simulink model "sampleModel1656"  (R2023a)
settings: Solver=VariableStepAuto  StartTime=0.0  StopTime=10.0  RelTol=1e-3
libraries: hdlsllib x6, simulink x1
settings Model: Creator=user1  LastModifiedBy=user1

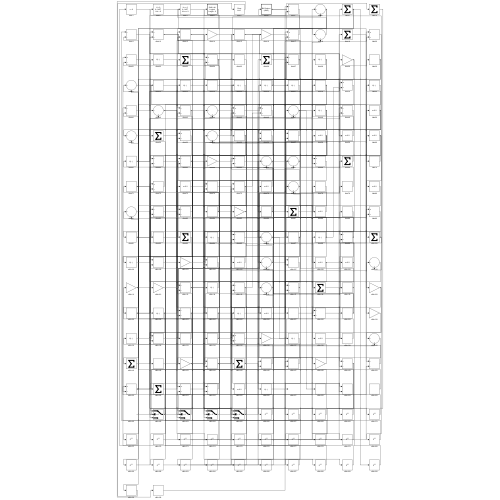
[thumbnail: Simulink's stored preview of the top-level diagram]
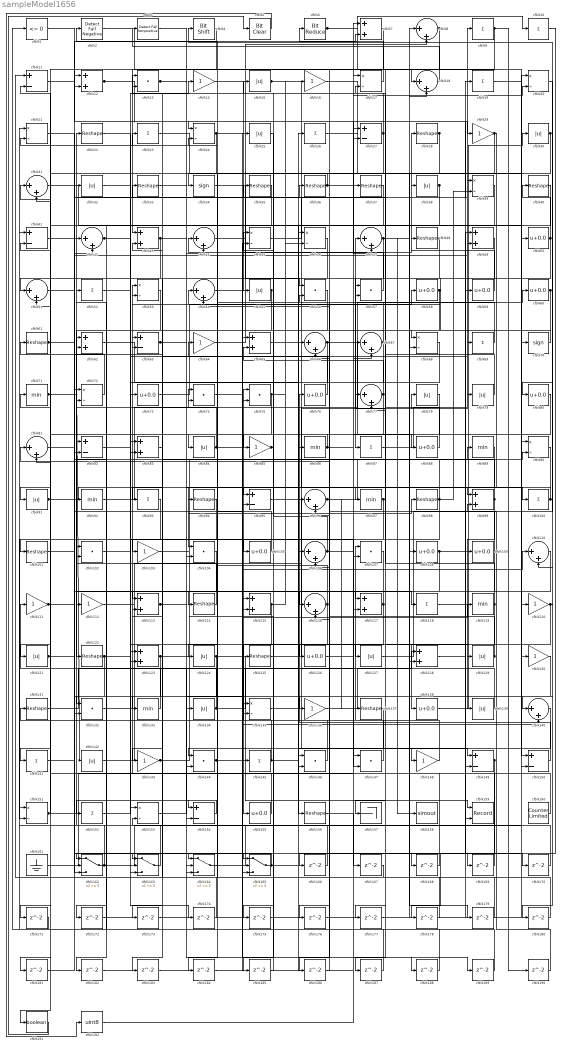
== system sampleModel1656 ==
  cfblk1 : hdlsllib/Logic and Bit Operations/Compare To Zero  relop=<=  OutDataTypeStr=boolean
  cfblk{9..10,19,23,26,52,69,87,93,100,118,141,145,152} (14 alike) : Sum  Inputs=+
  cfblk{22,28,33,35..37,40,48,61,94,98,101,114,122,125,131,137,156} (18 alike) : Reshape
  cfblk{13,56..57,74..75,102,104,107,132,144,146..147} (12 alike) : DotProduct  OutDataTypeStr=Inherit: Inherit via internal rule
  cfblk{14,16,29,64,85,103,111..112,120,130,136,143,148} (13 alike) : Gain
  cfblk{50,58..60,73,76,80,88,105,108..109,126,138,155} (14 alike) : Bias  Bias=0.0  SaturateOnIntegerOverflow=off
  cfblk{8,18,31,42,44,47,51,54,66..67,77,81,96,106,110,116,140} (17 alike) : Sum  Inputs=|++
  cfblk{11,27,41,63,82,95,149..150,154} (9 alike) : Sum  Inputs=+-
  cfblk{7,12,43,49,62,65,83,99,113,115,117,123,128} (13 alike) : Sum
  cfblk{71,86,89,92,97,119,133} (7 alike) : MinMax
  cfblk{15,25,30,32,38,55,78..79,84,91,121,124,127,129,134,139,142} (17 alike) : Abs  SaturateOnIntegerOverflow=off
  cfblk{17,20..21,24,39,45..46,53,68,72,90,135,151,153} (14 alike) : Product  Inputs=*/  RndMeth=Zero  SaturateOnIntegerOverflow=on
  cfblk157 : Terminator
  cfblk158 : ToWorkspace  VariableName=simout  SaveFormat=Timeseries  SampleTime=-1
  cfblk159 : Record  FileSettingsInternal="{\"entries\":[{\"content\":{\"excelSettings\":{\"content\":{},\"type\":\"Streamout.ExcelSettings\"}},\"type\":\"Streamout.FileSettingStorage\",\"uuid\":\"\"}],\"packageUris\":[\"http:\\/\\/schema.mathworks.com\\/mf0\\/streamout_blocks\\/R2020a\"],\"version\":\"1.0\"}"  Layout=[1 1]  SignalsInternal="{\"entries\":[{\"content\":{\"signals\":[{\"content\":{\"blockPath\":[],\"dimensions\":[1],\"domain\":\"\",\"lineColor\":\"#a2142f\",\"plots\":[1],\"port\":1,\"signalID\":2593,\"signalName\":\"XY Graph:1\"},\"type\":\"RecordBlkView.Signal\",\"uuid\":\"\"},{\"content\":{\"blockPath\":[],\"dimensions\":[1],\"domain\":\"\",\"lineColor\":\"#139fff\",\"plots\":[1],\"port\":2,\"signalID\":2596,\"signalName\":\"XY Graph:2\"},\"type\":\"RecordBlkView.Signal\",\"uuid\":\"\"}]},\"type\":\"RecordBlkView.InputSignals\",\"uuid\":\"\"}],\"packageUris\":[\"http:\\/\\/schema.mathworks.com\\/mf0\\/streamout_blocks\\/R2020a\"],\"version\":\"1.0\"}"  VisualizationBindings="{\"xyplotplugin\":{\"info\":[{\"series\":[{\"bindingParametersList\":[{\"parameter\":\"X-Axis\",\"signalID\":2593,\"signalName\":\"XY Graph:1\"},{\"parameter\":\"Y-Axis\",\"signalID\":2596,\"signalName\":\"XY Graph:2\"}],\"seriesID\":62182}],\"subplotID\":1}]}}"  CompatibilityTag=XY  st=-1
  cfblk160 : hdlsllib/Sources/Counter Limited  uplimit=7  tsamp=-1
  cfblk161 : Ground
  cfblk{162..165} (4 alike) : Switch  SaturateOnIntegerOverflow=off  InputSameDT=off
  cfblk{166..190} (25 alike) : Delay  SampleTime=1
  cfblk191 : DataTypeConversion  OutDataTypeStr=boolean  SaturateOnIntegerOverflow=off  RndMeth=Floor
  cfblk192 : DataTypeConversion  OutDataTypeStr=uint8  SaturateOnIntegerOverflow=off  RndMeth=Floor
  cfblk2 : hdlsllib/Logic and Bit Operations/Detect Fall Negative  vinit=0  OutDataTypeStr=boolean
  cfblk3 : hdlsllib/Logic and Bit Operations/Detect Fall Nonpositive  vinit=0  OutDataTypeStr=boolean
  cfblk34 : Signum
  cfblk4 : hdlsllib/Logic and Bit Operations/Bit Shift  mode=Shift Left Logical  N=0
  cfblk5 : simulink/Logic and Bit Operations/Bit Clear  iBit=0
      settings: LibrarySourceBlock=|
      | hdlsllib/Logic and Bit
      | Operations/Bit Clear
  cfblk6 : hdlsllib/Logic and Bit Operations/Bit Reduce  mode=AND
  cfblk70 : Signum
  wires:
  cfblk15/1 -> cfblk100/1, cfblk59/1
  cfblk13/1 -> cfblk165/1, cfblk189/1
  cfblk160/1 -> cfblk53/1
  cfblk150/1 -> cfblk76/1
  cfblk124/1 -> cfblk159/1, cfblk162/3
  cfblk103/1 -> cfblk98/1
  cfblk50/1 -> cfblk87/1, cfblk68/1, cfblk40/1, cfblk163/3
  cfblk59/1 -> cfblk28/1
  cfblk162/1 -> cfblk22/1, cfblk18/2
  cfblk46/1 -> cfblk103/1
  cfblk118/1 -> cfblk4/1
  cfblk101/1 -> cfblk12/1
  cfblk138/1 -> cfblk30/1
  cfblk143/1 -> cfblk89/1, cfblk125/1
  cfblk36/1 -> cfblk34/1, cfblk20/2
  cfblk149/1 -> cfblk177/1, cfblk178/1
  cfblk148/1 -> cfblk107/1
  cfblk125/1 -> cfblk78/1
  cfblk6/1 -> cfblk10/1, cfblk18/1
  cfblk127/1 -> cfblk50/1
  cfblk27/1 -> cfblk144/1, cfblk96/2, cfblk13/2
  cfblk142/1 -> cfblk66/1
  cfblk73/1 -> cfblk58/1
  cfblk41/1 -> cfblk12/2
  cfblk71/1 -> cfblk142/1, cfblk118/1
  cfblk55/1 -> cfblk122/1, cfblk163/1
  cfblk20/1 -> cfblk80/1
  cfblk19/1 -> cfblk70/1
  cfblk104/1 -> cfblk114/1
  cfblk96/1 -> cfblk20/1, cfblk137/1
  cfblk113/1 -> cfblk127/1, cfblk165/2
  cfblk120/1 -> cfblk138/1, cfblk180/1
  cfblk9/1 -> cfblk43/1, cfblk117/1, cfblk190/1
  cfblk163/1 -> cfblk52/1
  cfblk91/1 -> cfblk97/1, cfblk95/2
  cfblk64/1 -> cfblk8/2
  cfblk161/1 -> cfblk73/1
  cfblk95/1 -> cfblk148/1
  cfblk76/1 -> cfblk23/1
  cfblk117/1 -> cfblk112/1, cfblk185/1
  cfblk21/1 -> cfblk42/1
  cfblk147/1 -> cfblk75/1
  cfblk99/1 -> cfblk139/1, cfblk45/1, cfblk63/2
  cfblk112/1 -> cfblk60/1
  cfblk53/1 -> cfblk62/1
  cfblk116/1 -> cfblk155/1, cfblk74/2
  cfblk58/1 -> cfblk53/2, cfblk164/1, cfblk68/2, cfblk164/3
  cfblk67/1 -> cfblk2/1, cfblk124/1
  cfblk87/1 -> cfblk9/1
  cfblk31/1 -> cfblk150/1
  cfblk102/1 -> cfblk126/1
  cfblk25/1 -> cfblk85/1
  cfblk132/1 -> cfblk79/1
  cfblk42/1 -> cfblk153/1, cfblk107/2
  cfblk23/1 -> cfblk120/1
  cfblk57/1 -> cfblk44/1
  cfblk51/1 -> cfblk49/2
  cfblk98/1 -> cfblk147/2, cfblk77/1, cfblk66/2, cfblk39/2
  cfblk47/1 -> cfblk162/2, cfblk158/1, cfblk179/1
  cfblk12/1 -> cfblk55/1, cfblk47/2
  cfblk79/1 -> cfblk54/1
  cfblk65/1 -> cfblk86/1
  cfblk61/1 -> cfblk38/1, cfblk7/2
  cfblk24/1 -> cfblk21/2, cfblk82/2, cfblk140/2
  cfblk137/1 -> cfblk154/1
  cfblk17/1 -> cfblk6/1
  cfblk133/1 -> cfblk111/1
  cfblk11/1 -> cfblk29/1
  cfblk3/1 -> cfblk44/2
  cfblk8/1 -> cfblk136/1, cfblk51/2
  cfblk33/1 -> cfblk116/1
  cfblk121/1 -> cfblk33/1, cfblk63/1
  cfblk134/1 -> cfblk61/1, cfblk67/2
  cfblk153/1 -> cfblk134/1
  cfblk152/1 -> cfblk69/1
  cfblk89/1 -> cfblk104/1
  cfblk83/1 -> cfblk13/1
  cfblk135/1 -> cfblk149/1
  cfblk44/1 -> cfblk156/1
  cfblk52/1 -> cfblk14/1
  cfblk34/1 -> cfblk96/1
  cfblk62/1 -> cfblk106/1
  cfblk164/1 -> cfblk90/1
  cfblk86/1 -> cfblk84/1, cfblk88/1
  cfblk30/1 -> cfblk105/1, cfblk51/1
  cfblk4/1 -> cfblk101/1
  cfblk92/1 -> cfblk47/1
  cfblk88/1 -> cfblk32/1
  cfblk115/1 -> cfblk145/1, cfblk46/2
  cfblk16/1 -> cfblk149/2
  cfblk82/1 -> cfblk123/1
  cfblk131/1 -> cfblk17/1
  cfblk151/1 -> cfblk27/1, cfblk90/2, cfblk31/2
  cfblk136/1 -> cfblk128/1
  cfblk154/1 -> cfblk152/1
  cfblk32/1 -> cfblk83/1
  cfblk1/1 -> cfblk24/1
  cfblk69/1 -> cfblk17/2
  cfblk56/1 -> cfblk113/1
  cfblk105/1 -> cfblk74/1
  cfblk90/1 -> cfblk154/2
  cfblk77/1 -> cfblk92/1, cfblk65/2
  cfblk84/1 -> cfblk62/2, cfblk188/1
  cfblk68/1 -> cfblk83/2
  cfblk66/1 -> cfblk108/1, cfblk143/1
  cfblk49/1 -> cfblk133/1
  cfblk28/1 -> cfblk57/1, cfblk164/2
  cfblk122/1 -> cfblk36/1, cfblk132/2
  cfblk72/1 -> cfblk11/2
  cfblk119/1 -> cfblk157/1, cfblk77/2
  cfblk129/1 -> cfblk81/1, cfblk64/1
  cfblk37/1 -> cfblk81/2
  cfblk48/1 -> cfblk104/2, cfblk163/2, cfblk191/1
  cfblk146/1 -> cfblk71/1
  cfblk97/1 -> cfblk57/2, cfblk121/1, cfblk151/2
  cfblk109/1 -> cfblk54/2, cfblk117/2
  cfblk106/1 -> cfblk39/1, cfblk35/1
  cfblk7/1 -> cfblk56/1
  cfblk14/1 -> cfblk25/1
  cfblk45/1 -> cfblk19/1
  cfblk126/1 -> cfblk7/1
  cfblk111/1 -> cfblk41/2, cfblk165/3
  cfblk141/1 -> cfblk72/1
  cfblk2/1 -> cfblk130/1
  cfblk26/1 -> cfblk128/2
  cfblk43/1 -> cfblk91/1, cfblk168/1
  cfblk114/1 -> cfblk82/1
  cfblk165/1 -> cfblk26/1, cfblk162/1
  cfblk85/1 -> cfblk15/1, cfblk135/1
  cfblk35/1 -> cfblk132/1
  cfblk60/1 -> cfblk110/2, cfblk182/1, cfblk183/1
  cfblk39/1 -> cfblk146/2
  cfblk155/1 -> cfblk31/1
  cfblk18/1 -> cfblk3/1
  cfblk94/1 -> cfblk141/1
  cfblk144/1 -> cfblk119/1, cfblk110/1
  cfblk63/1 -> cfblk93/1, cfblk135/2
  cfblk54/1 -> cfblk48/1
  cfblk29/1 -> cfblk99/1, cfblk123/2
  cfblk75/1 -> cfblk102/1, cfblk16/1
  cfblk40/1 -> cfblk144/2
  cfblk108/1 -> cfblk109/1, cfblk186/1
  cfblk100/1 -> cfblk95/1, cfblk140/1
  cfblk123/1 -> cfblk45/2, cfblk172/1
  cfblk70/1 -> cfblk67/1
  cfblk139/1 -> cfblk115/1
  cfblk145/1 -> cfblk159/2, cfblk131/1
  cfblk74/1 -> cfblk129/1
  cfblk38/1 -> cfblk94/1, cfblk116/2
  cfblk10/1 -> cfblk166/1
  cfblk166/1 -> cfblk21/1
  cfblk156/1 -> cfblk167/1
  cfblk167/1 -> cfblk11/1
  cfblk168/1 -> cfblk56/2
  cfblk81/1 -> cfblk169/1
  cfblk169/1 -> cfblk43/2
  cfblk128/1 -> cfblk170/1
  cfblk170/1 -> cfblk153/2
  cfblk80/1 -> cfblk171/1
  cfblk171/1 -> cfblk1/1
  cfblk172/1 -> cfblk75/2
  cfblk130/1 -> cfblk173/1
  cfblk173/1 -> cfblk150/2
  cfblk22/1 -> cfblk174/1
  cfblk174/1 -> cfblk113/2
  cfblk107/1 -> cfblk175/1
  cfblk175/1 -> cfblk49/1
  cfblk140/1 -> cfblk176/1
  cfblk176/1 -> cfblk147/1
  cfblk177/1 -> cfblk8/1
  cfblk178/1 -> cfblk72/2
  cfblk179/1 -> cfblk41/1
  cfblk180/1 -> cfblk24/2
  cfblk93/1 -> cfblk181/1
  cfblk181/1 -> cfblk42/2
  cfblk182/1 -> cfblk65/1
  cfblk183/1 -> cfblk27/2
  cfblk110/1 -> cfblk184/1
  cfblk184/1 -> cfblk46/1
  cfblk185/1 -> cfblk115/2
  cfblk186/1 -> cfblk106/2
  cfblk78/1 -> cfblk187/1
  cfblk187/1 -> cfblk146/1
  cfblk188/1 -> cfblk102/2
  cfblk189/1 -> cfblk151/1
  cfblk190/1 -> cfblk99/2
  cfblk191/1 -> cfblk5/1
  cfblk5/1 -> cfblk192/1
  cfblk192/1 -> cfblk37/1
